simulink model "regWaveNLYawTest"  (R2019a)
settings: Solver=ode4  StartTime=0.0  StopTime=1200  FixedStep=0.01  RelTol=1e-3
values from neighbouring files (symbols this model uses):
  simu = simulationClass()    [wecSimInputFile.m]
  waves = waveClass('regular')    [wecSimInputFile.m]
undefined symbols (not defined in the file or in its folder): body
libraries: simulink x1
settings Model: Creator=dforbus  LastModifiedBy=dforbus

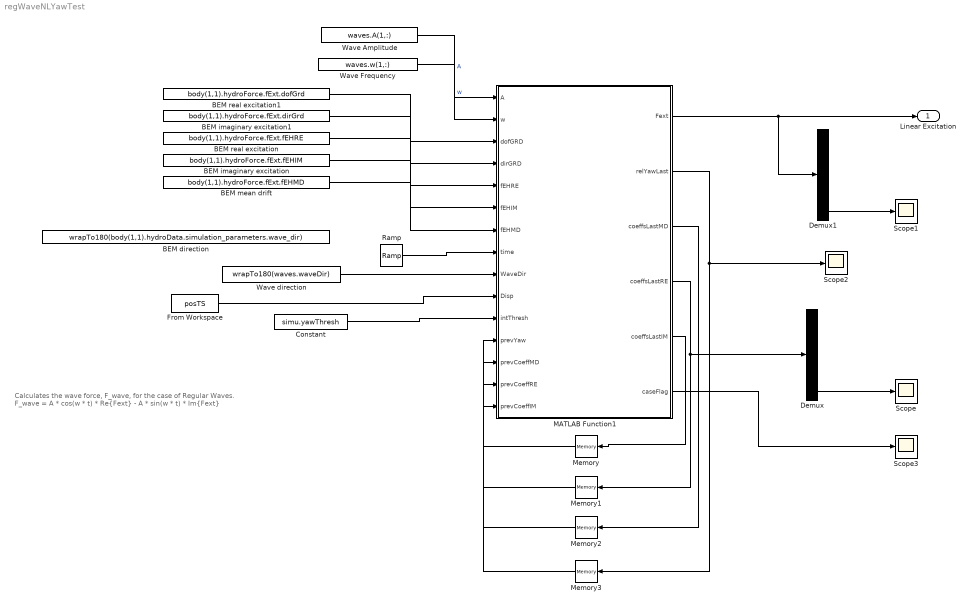
== system regWaveNLYawTest ==
  note: Calculates the wave force, F_wave, for the case of Regular Waves.
      |
      | F_wave =   A * cos(w * t) * Re{Fext}
      |                -  A * sin(w * t) * Im{Fext}
  BEM direction : Constant  Value=wrapTo180(body(1,1).hydroData.simulation_parameters.wave_dir)  VectorParams1D=off
  BEM imaginary excitation : Constant  Value=body(1,1).hydroForce.fExt.fEHIM  VectorParams1D=off
  BEM imaginary excitation1 : Constant  Value=body(1,1).hydroForce.fExt.dirGrd  VectorParams1D=off
  BEM mean drift : Constant  Value=body(1,1).hydroForce.fExt.fEHMD  VectorParams1D=off
  BEM real excitation : Constant  Value=body(1,1).hydroForce.fExt.fEHRE  VectorParams1D=off
  BEM real excitation1 : Constant  Value=body(1,1).hydroForce.fExt.dofGrd  VectorParams1D=off
  Constant : Constant  Value=simu.yawThresh
  Demux : Demux  Outputs=6
  Demux1 : Demux  Outputs=6
  From Workspace : FromWorkspace  VariableName=posTS
  MATLAB Function1 : MATLAB Function  AncestorBlock=|  TreatAsAtomicUnit=on
      | WECSim_Lib/Body Elements/Rigid Body/Hydrodynamic Body/Wave Diffraction and Excitation Force Calculation/Linear Wave Excitation Force Variant Subsystem/Regular Wave
      | NonLinear Yaw/MATLAB Function1
  Memory{,1..3} (4 alike) : Memory  InheritSampleTime=on  LinearizeAsDelay=on
  Ramp : simulink/Sources/Ramp  slope=1  start=0  InitialOutput=0
  Scope{,1..3} (4 alike) : Scope
  Wave Amplitude : Constant  Value=waves.A(1,:)
  Wave Frequency : Constant  Value=waves.w(1,:)
  Wave direction : Constant  Value=wrapTo180(waves.waveDir)  VectorParams1D=off
  Linear Excitation : Outport
  wires:
  BEM imaginary excitation/1 -> MATLAB Function1/6(fEHIM)
  Constant/1 -> MATLAB Function1/11(intThresh)
  From Workspace/1 -> MATLAB Function1/10(Disp)
  BEM real excitation1/1 -> MATLAB Function1/3(dofGRD)
  MATLAB Function1/3(coeffsLastMD) -> Memory2/1
  MATLAB Function1/1(Fext) -> Demux1/1, Linear Excitation/1
  Wave direction/1 -> MATLAB Function1/9(WaveDir)
  Memory1/1 -> MATLAB Function1/14(prevCoeffRE)
  Ramp/1 -> MATLAB Function1/8(time)
  BEM real excitation/1 -> MATLAB Function1/5(fEHRE)
  BEM imaginary excitation1/1 -> MATLAB Function1/4(dirGRD)
  Memory2/1 -> MATLAB Function1/13(prevCoeffMD)
  Wave Amplitude/1 -> MATLAB Function1/1(A)  "A"
  Memory/1 -> MATLAB Function1/15(prevCoeffIM)
  Memory3/1 -> MATLAB Function1/12(prevYaw)
  MATLAB Function1/5(coeffsLastIM) -> Memory/1
  Wave Frequency/1 -> MATLAB Function1/2(w)  "w"
  MATLAB Function1/2(relYawLast) -> Scope2/1, Memory3/1
  BEM mean drift/1 -> MATLAB Function1/7(fEHMD)
  MATLAB Function1/4(coeffsLastRE) -> Demux/1, Memory1/1
  Demux/6 -> Scope/1
  Demux1/6 -> Scope1/1
  MATLAB Function1/6(caseFlag) -> Scope3/1

== matlab function regWaveNLYawTest/MATLAB Function1 ==
  data: A input; w input; dofGRD input; dirGRD input; fEHRE input; fEHIM input; Fext output; fEHMD input; time input; WaveDir input; Disp input; intThresh input; prevYaw input; relYawLast output; prevCoeffMD input; prevCoeffRE input; prevCoeffIM input; coeffsLastMD output; coeffsLastRE output; coeffsLastIM output; caseFlag output
function [Fext,relYawLast,coeffsLastMD,coeffsLastRE,coeffsLastIM, caseFlag] = fcn(A,w,dofGRD,dirGRD,fEHRE,fEHIM, fEHMD,time,WaveDir,Disp, intThresh, prevYaw, prevCoeffMD, prevCoeffRE, prevCoeffIM)
%#codegen
% Fext is the excitation force output, relYawLast is the angle of relative
% yaw at which that last interpolation was performed. If the current
% relative yaw angle - last interpolated > threshold, the interpolation is
% performed again. To interpolate every time step, let threshold=0. 


%initialize outputs
Fext = zeros(1,6);
relYawLast=0;
coeffsLastMD=zeros(length(w),6); % should be (1,6) for regular waves
coeffsLastRE=zeros(length(w),6);
coeffsLastIM=zeros(length(w),6);

for ii=1:length(WaveDir) % should be length=1 for regular waves
    relYaw=WaveDir(ii)-(Disp.*180/pi); % relative yaw angle, convert to deg
   
    % compare relYaw to available WaveDir data
        if relYaw>max(dirGRD(1,:)) % handle interpolation out of BEM range by wrapping other bound
            [~,idx]=min(dirGRD,[],2); % 
            dirGRD(:,idx)=dirGRD(:,idx)+360;
            [dirGRD,I]=sort(dirGRD,2); % grid must be in ascending order
            
        elseif relYaw<min(dirGRD(1,:))
            [~,idx]=max(dirGRD,[],2); % 
            dirGRD(:,idx)=dirGRD(:,idx)-360;
            [dirGRD,I]=sort(dirGRD,2); % grid must be in ascending order
        else
            I=1:length(dirGRD(1,:));
            
        end
    
    if abs(relYaw-prevYaw)>intThresh && min(abs(relYaw-dirGRD(1,:)))>intThresh% interpolate for nonlinear yaw 
        
        % performs 1D interpolation in wave direction
        fExtMDint=interpn(dofGRD,dirGRD,fEHMD(:,I(1,:)),dofGRD,relYaw*ones(size(dirGRD)));
        fExtREint=interpn(dofGRD,dirGRD,fEHRE(:,I(1,:)),dofGRD,relYaw*ones(size(dirGRD)));
        fExtIMint=interpn(dofGRD,dirGRD,fEHIM(:,I(1,:)),dofGRD,relYaw*ones(size(dirGRD)));
        
        fExtMDint=fExtMDint(:,1).';
        fExtREint=fExtREint(:,1).';
        fExtIMint=fExtIMint(:,1).';
                
        relYawLast=relYaw;
        coeffsLastMD=fExtMDint;
        coeffsLastRE=fExtREint;
        coeffsLastIM=fExtIMint;
        
        caseFlag=1;
  
    elseif min(abs(relYaw-dirGRD(1,:)))>intThresh % significant yaw is present, but close to previous value
        fExtMDint=prevCoeffMD;
        fExtREint=prevCoeffRE;
        fExtIMint=prevCoeffIM;
        
        relYawLast=prevYaw;
        coeffsLastMD=prevCoeffMD;
        coeffsLastRE=prevCoeffRE;
        coeffsLastIM=prevCoeffIM;
        
        caseFlag=2;
      
    else    % significant yaw may be is present, but nearby pre-calculated data
        [~,idx]=min(abs(relYaw-dirGRD(1,:)));
        fExtMDint=fEHMD(:,I(1,idx)).'; % maintains dimensional consistency
        fExtREint=fEHRE(:,I(1,idx)).';
        fExtIMint=fEHIM(:,I(1,idx)).';
     
        relYawLast=dirGRD(1,idx); % indices of dirGRD have already been resorted
        coeffsLastMD=fExtMDint;
        coeffsLastRE=fExtREint;
        coeffsLastIM=fExtIMint;
        
        caseFlag=3;
    
    end

    % regular wave excitation equation (with mean drift)
    Fext = fExtMDint*A^2 + A*fExtREint*cos(w*time)- A*fExtIMint*sin(w*time);
end
